simulink model "ball_on_beam_subsystem"  (R2025b)
settings: Solver=VariableStepAuto  StartTime=0.0  StopTime=20.0  MaxStep=1e-3  RelTol=1e-3
values from neighbouring files (symbols this model uses):
  c = Simulink.Parameter    [motorised_BoB_system_with_PID.m]
  g = Simulink.Parameter    [motorised_BoB_system_with_PID.m]
  KDpid = Simulink.Parameter    [motorised_BoB_system_with_PID.m]
  KIpid = Simulink.Parameter    [motorised_BoB_system_with_PID.m]
  KPpid = Simulink.Parameter    [motorised_BoB_system_with_PID.m]
settings Model: Creator=fycce  LastModifiedBy=fycce

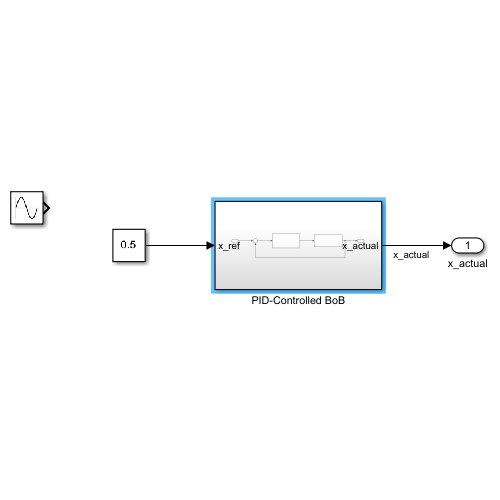
[thumbnail: Simulink's stored preview of the top-level diagram]
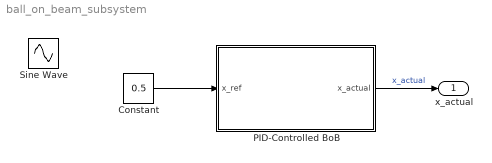
== system ball_on_beam_subsystem ==
  Constant : Constant  Value=0.5
  PID-Controlled BoB : Subsystem
  Sine Wave : Sin  Amplitude=0.25  Frequency=pi/2  SampleTime=0
  x_actual : Outport
  wires:
  PID-Controlled BoB/1(x_actual) -> x_actual/1  "x_actual"
  Constant/1 -> PID-Controlled BoB/1(x_ref)

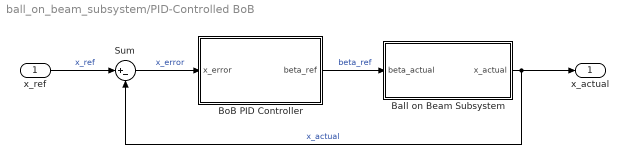
== system ball_on_beam_subsystem/PID-Controlled BoB ==
  x_ref : Inport
  Ball on Beam Subsystem : Subsystem
  BoB PID Controller : Subsystem
  Sum : Sum  Inputs=|+-
  x_actual : Outport
  wires:
  Sum/1 -> BoB PID Controller/1(x_error)  "x_error"
  BoB PID Controller/1(beta_ref) -> Ball on Beam Subsystem/1(beta_actual)  "beta_ref"
  Ball on Beam Subsystem/1(x_actual) -> x_actual/1, Sum/2  "x_actual"
  x_ref/1 -> Sum/1  "x_ref"

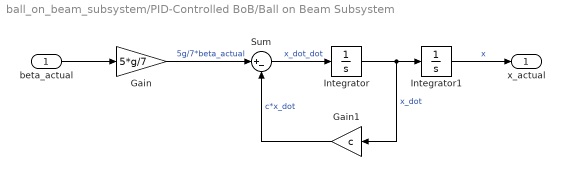
== system ball_on_beam_subsystem/PID-Controlled BoB/Ball on Beam Subsystem ==
  beta_actual : Inport
  Gain : Gain  Gain=5*g/7
  Gain1 : Gain  Gain=c
  Integrator : Integrator
  Integrator1 : Integrator
  Sum : Sum  Inputs=|+-
  x_actual : Outport
  wires:
  Integrator1/1 -> x_actual/1  "x"
  beta_actual/1 -> Gain/1
  Integrator/1 -> Integrator1/1, Gain1/1  "x_dot"
  Sum/1 -> Integrator/1  "x_dot_dot"
  Gain1/1 -> Sum/2  "c*x_dot"
  Gain/1 -> Sum/1  "5g/7*beta_actual"

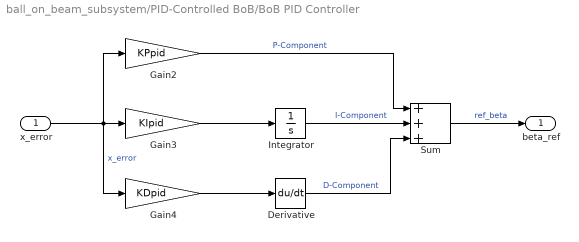
== system ball_on_beam_subsystem/PID-Controlled BoB/BoB PID Controller ==
  x_error : Inport
  Derivative : Derivative
  Gain2 : Gain  Gain=KPpid
  Gain3 : Gain  Gain=KIpid
  Gain4 : Gain  Gain=KDpid
  Integrator : Integrator
  Sum : Sum  Inputs=+++
  beta_ref : Outport
  wires:
  Gain4/1 -> Derivative/1
  Derivative/1 -> Sum/3  "D-Component"
  Sum/1 -> beta_ref/1  "ref_beta"
  Integrator/1 -> Sum/2  "I-Component"
  Gain3/1 -> Integrator/1
  x_error/1 -> Gain4/1, Gain3/1, Gain2/1  "x_error"
  Gain2/1 -> Sum/1  "P-Component"
